simulink model "simulinkModel"  (R2015a)
settings: Solver=ode45  StartTime=0.0  StopTime=10.0  RelTol=1e-3
values from neighbouring files (symbols this model uses):
  CL0 = 0    [loadModel_EB.m]
  CLa = 22    [loadModel_EB.m]
  Cm0 = 0    [loadModel_EB.m]
  Cma = 75    [loadModel_EB.m]
  g = [gx;gextra]    [getRigidBodySS.m]
  m = sum(dm)    [getRigidBodySS.m]
  rho = 1.21    [loadModel_EB.m]
  theta0 = double(theta0)    [getRigidBodySS.m]
  xCM = (1-0.84)*total_length    (= 0.784)    [loadModel_EB.m]
undefined symbols (not defined in the file or in its folder): gamma0, ICG, Lref, Sref, theta_dot0, V0, x0, xCG, z0
libraries: simulink_extras x2, aerolib3dof2 x1, aerolibasang x1
settings Model: Creator=anatole  LastModifiedBy=anatole

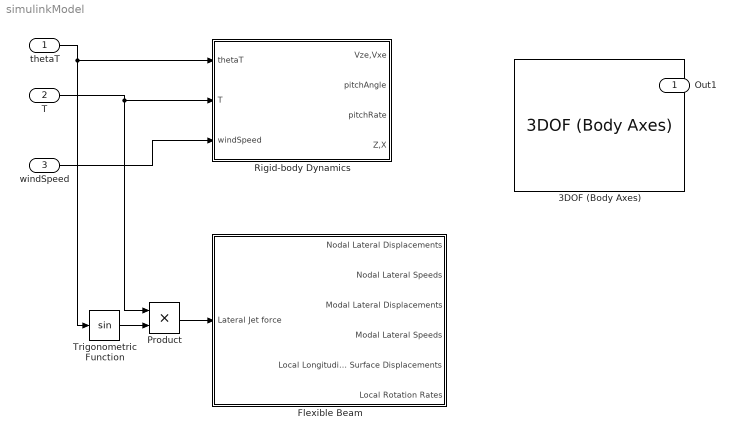
== system simulinkModel ==
  thetaT : Inport
  T : Inport  Port=2
  windSpeed : Inport  Port=3
  3DOF (Body Axes) : aerolib3dof2/3DOF (Body Axes)  units=Metric (MKS)  mtype=Fixed  v_ini=100  theta_ini=0  alpha_ini=0  q_ini=0  pos_ini=[0 0]  mass=1.0  mass_e=0.5  mass_f=3.0  Iyy=1.0  Iyy_e=0.5  Iyy_f=3.0  g_in=External  g=9.81  vre_flag=on
  Flexible Beam : Subsystem
  Product : Product
  Rigid-body Dynamics : Subsystem
  Trigonometric Function : Trigonometry
  Out1 : Outport
  wires:
  T/1 -> Product/1, Rigid-body Dynamics/2(T)
  thetaT/1 -> Trigonometric Function/1, Rigid-body Dynamics/1(thetaT)
  windSpeed/1 -> Rigid-body Dynamics/3(windSpeed)
  Product/1 -> Flexible Beam/1(Lateral Jet force)
  Trigonometric Function/1 -> Product/2

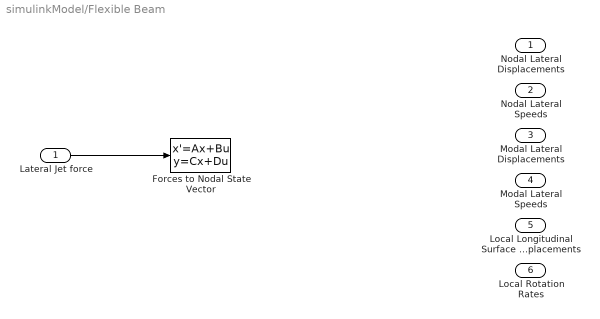
== system simulinkModel/Flexible Beam ==
  Lateral Jet force : Inport
  Forces to Nodal State Vector : StateSpace  X0=0
  Nodal Lateral Displacements : Outport
  Nodal Lateral Speeds : Outport  Port=2
  Modal Lateral Displacements : Outport  Port=3
  Modal Lateral Speeds : Outport  Port=4
  Local Longitudinal Surface Displacements : Outport  Port=5
  Local Rotation Rates : Outport  Port=6
  wires:
  Lateral Jet force/1 -> Forces to Nodal State Vector/1

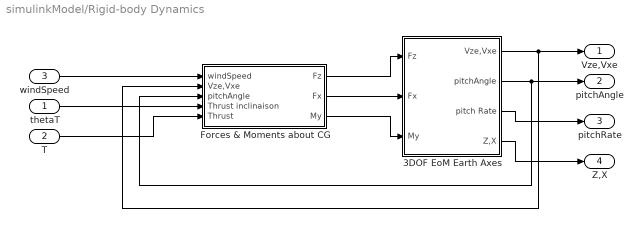
== system simulinkModel/Rigid-body Dynamics ==
  thetaT : Inport
  T : Inport  Port=2
  windSpeed : Inport  Port=3
  3DOF EoM Earth Axes : Subsystem
  Forces & Moments about CG : Subsystem
  Vze,Vxe : Outport
  pitchAngle : Outport  Port=2
  pitchRate : Outport  Port=3
  Z,X : Outport  Port=4
  wires:
  windSpeed/1 -> Forces & Moments about CG/1(windSpeed)
  3DOF EoM Earth Axes/1(Vze,Vxe) -> Forces & Moments about CG/2(Vze,Vxe), Vze,Vxe/1
  3DOF EoM Earth Axes/2(pitchAngle) -> pitchAngle/1, Forces & Moments about CG/3(pitchAngle)
  thetaT/1 -> Forces & Moments about CG/4(Thrust inclinaison)
  T/1 -> Forces & Moments about CG/5(Thrust)
  Forces & Moments about CG/3("My ") -> 3DOF EoM Earth Axes/3(My)
  Forces & Moments about CG/1(Fz) -> 3DOF EoM Earth Axes/1(Fz)
  Forces & Moments about CG/2(Fx) -> 3DOF EoM Earth Axes/2(Fx)
  3DOF EoM Earth Axes/3(pitch Rate) -> pitchRate/1
  3DOF EoM Earth Axes/4(Z,X) -> Z,X/1

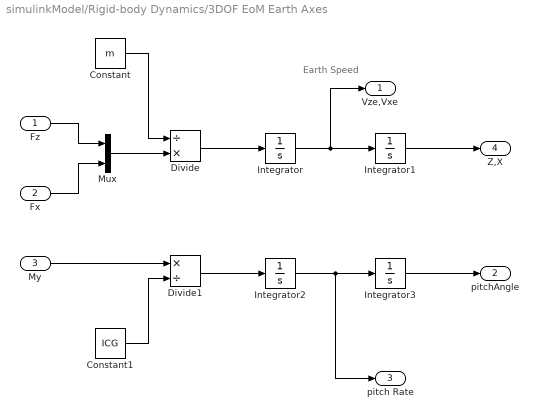
== system simulinkModel/Rigid-body Dynamics/3DOF EoM Earth Axes ==
  note: Earth Speed
  Fz : Inport
  Fx : Inport  Port=2
  My : Inport  Port=3
  Constant : Constant  Value=m
  Constant1 : Constant  Value=ICG
  Divide : Product  Inputs=/*
  Divide1 : Product  Inputs=*/
  Integrator : Integrator  InitialCondition=[-V0*sin(gamma0), V0*cos(gamma0)]
  Integrator1 : Integrator  InitialCondition=[z0, x0]
  Integrator2 : Integrator  InitialCondition=theta_dot0
  Integrator3 : Integrator  InitialCondition=theta0
  Mux : Mux  Inputs=2
  Vze,Vxe : Outport
  pitchAngle : Outport  Port=2
  pitch Rate : Outport  Port=3
  Z,X : Outport  Port=4
  wires:
  Fz/1 -> Mux/1
  Fx/1 -> Mux/2
  Mux/1 -> Divide/2
  Constant/1 -> Divide/1
  Divide/1 -> Integrator/1
  Integrator/1 -> Vze,Vxe/1, Integrator1/1
  My/1 -> Divide1/1
  Constant1/1 -> Divide1/2
  Integrator2/1 -> pitch Rate/1, Integrator3/1
  Divide1/1 -> Integrator2/1
  Integrator3/1 -> pitchAngle/1
  Integrator1/1 -> Z,X/1

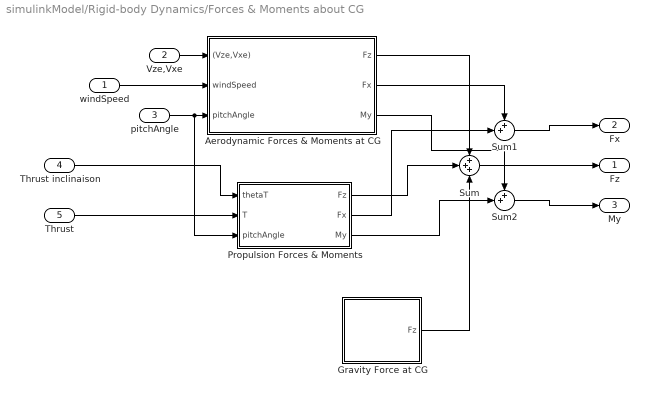
== system simulinkModel/Rigid-body Dynamics/Forces & Moments about CG ==
  windSpeed : Inport
  Vze,Vxe : Inport  Port=2
  pitchAngle : Inport  Port=3
  Thrust inclinaison : Inport  Port=4
  Thrust : Inport  Port=5
  Aerodynamic Forces & Moments at CG : Subsystem
  Gravity Force at CG : Subsystem
  Propulsion Forces & Moments : Subsystem
  Sum : Sum  Inputs=+++
  Sum1 : Sum  Inputs=++|
  Sum2 : Sum  Inputs=++|
  Fz : Outport
  Fx : Outport  Port=2
  "My " : Outport  Port=3
  wires:
  pitchAngle/1 -> Propulsion Forces & Moments/3(pitchAngle), Aerodynamic Forces & Moments at CG/3(pitchAngle)
  Propulsion Forces & Moments/3(My) -> Sum2/2
  Propulsion Forces & Moments/1(Fz) -> Sum/2
  windSpeed/1 -> Aerodynamic Forces & Moments at CG/2(windSpeed)
  Vze,Vxe/1 -> Aerodynamic Forces & Moments at CG/1((Vze,Vxe))
  Gravity Force at CG/1(Fz) -> Sum/3
  Propulsion Forces & Moments/2(Fx) -> Sum1/2
  Aerodynamic Forces & Moments at CG/3(My) -> Sum2/1
  Thrust/1 -> Propulsion Forces & Moments/2(T)
  Aerodynamic Forces & Moments at CG/1(Fz) -> Sum/1
  Aerodynamic Forces & Moments at CG/2(Fx) -> Sum1/1
  Sum/1 -> Fz/1
  Sum2/1 -> "My "/1
  Sum1/1 -> Fx/1
  Thrust inclinaison/1 -> Propulsion Forces & Moments/1(thetaT)

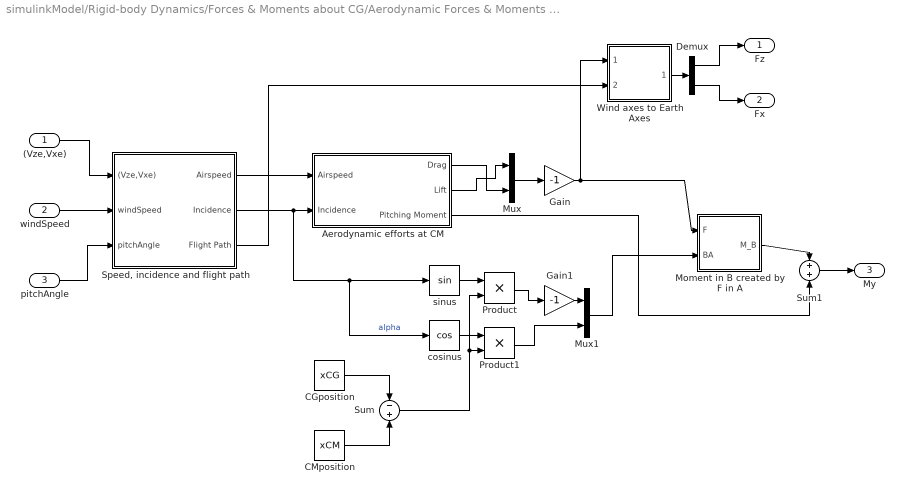
== system simulinkModel/Rigid-body Dynamics/Forces & Moments about CG/Aerodynamic Forces & Moments at CG ==
  (Vze,Vxe) : Inport
  windSpeed : Inport  Port=2
  pitchAngle : Inport  Port=3
  Aerodynamic efforts at CM : Subsystem
  CGposition : Constant  Value=xCG
  CMposition : Constant  Value=xCM
  Demux : Demux  Outputs=2
  Gain : Gain  Gain=-1
  Gain1 : Gain  Gain=-1
  Moment in B created by F in A : Subsystem
  Mux : Mux  Inputs=2
  Mux1 : Mux  Inputs=2
  Product : Product
  Product1 : Product
  "Speed, incidence and flight path" : Subsystem
  Sum : Sum  Inputs=-+
  Sum1 : Sum
  Wind axes to Earth Axes : Subsystem
  cosinus : Trigonometry  Operator=cos
  sinus : Trigonometry
  Fz : Outport
  Fx : Outport  Port=2
  My : Outport  Port=3
  wires:
  windSpeed/1 -> "Speed, incidence and flight path"/2(windSpeed)
  (Vze,Vxe)/1 -> "Speed, incidence and flight path"/1((Vze,Vxe))
  pitchAngle/1 -> "Speed, incidence and flight path"/3(pitchAngle)
  "Speed, incidence and flight path"/1(Airspeed) -> Aerodynamic efforts at CM/1(Airspeed)
  "Speed, incidence and flight path"/2(Incidence) -> cosinus/1, sinus/1, Aerodynamic efforts at CM/2(Incidence)  "alpha"
  Aerodynamic efforts at CM/2(Lift) -> Mux/1
  Aerodynamic efforts at CM/1(Drag) -> Mux/2
  Mux/1 -> Gain/1
  CGposition/1 -> Sum/1
  CMposition/1 -> Sum/2
  sinus/1 -> Product/1
  cosinus/1 -> Product1/1
  Sum/1 -> Product/2, Product1/2
  Product1/1 -> Mux1/2
  Product/1 -> Gain1/1
  Gain1/1 -> Mux1/1
  Mux1/1 -> Moment in B created by F in A/2(BA)
  Gain/1 -> Moment in B created by F in A/1(F), Wind axes to Earth Axes/1(vec_w)
  Sum1/1 -> My/1
  Aerodynamic efforts at CM/3(Pitching Moment) -> Sum1/2
  Moment in B created by F in A/1(M_B) -> Sum1/1
  "Speed, incidence and flight path"/3(Flight Path) -> Wind axes to Earth Axes/2(gamma)
  Wind axes to Earth Axes/1(vec_e) -> Demux/1
  Demux/1 -> Fz/1
  Demux/2 -> Fx/1

== system simulinkModel/Rigid-body Dynamics/Forces & Moments about CG/Gravity Force at CG ==
  Constant : Constant  Value=m*g
  Fz : Outport
  wires:
  Constant/1 -> Fz/1

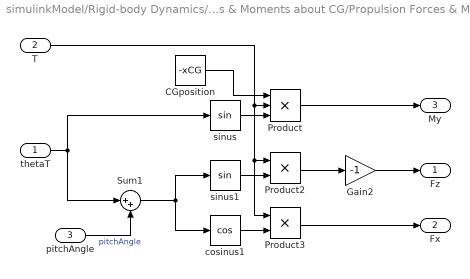
== system simulinkModel/Rigid-body Dynamics/Forces & Moments about CG/Propulsion Forces & Moments ==
  thetaT : Inport
  T : Inport  Port=2
  pitchAngle : Inport  Port=3
  CGposition : Constant  Value=-xCG
  Gain2 : Gain  Gain=-1
  Product : Product  Inputs=3
  Product2 : Product
  Product3 : Product
  Sum1 : Sum  Inputs=|++
  cosinus1 : Trigonometry  Operator=cos
  sinus : Trigonometry
  sinus1 : Trigonometry
  Fz : Outport
  Fx : Outport  Port=2
  My : Outport  Port=3
  wires:
  pitchAngle/1 -> Sum1/2  "pitchAngle"
  CGposition/1 -> Product/1
  T/1 -> Product/2, Product3/1, Product2/1
  sinus1/1 -> Product2/2
  cosinus1/1 -> Product3/2
  thetaT/1 -> sinus/1, Sum1/1
  Sum1/1 -> cosinus1/1, sinus1/1
  Product2/1 -> Gain2/1
  Gain2/1 -> Fz/1
  Product3/1 -> Fx/1
  sinus/1 -> Product/3
  Product/1 -> My/1

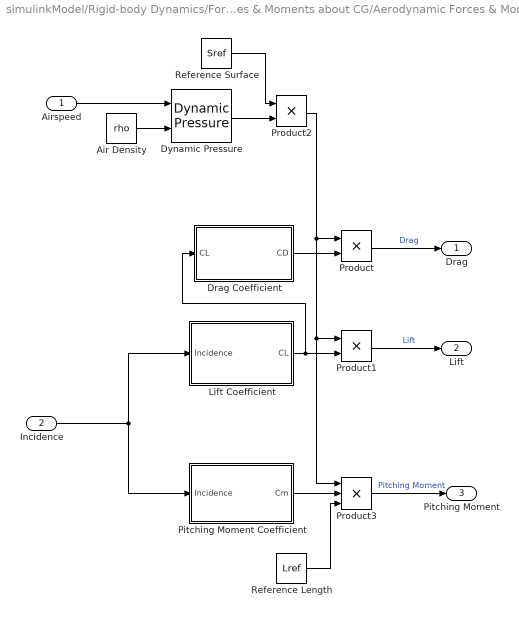
== system simulinkModel/Rigid-body Dynamics/Forces & Moments about CG/Aerodynamic Forces & Moments at CG/Aerodynamic efforts at CM ==
  Airspeed : Inport
  Incidence : Inport  Port=2
  Air Density : Constant  Value=rho
  Drag Coefficient : Subsystem
  Dynamic Pressure : aerolibasang/Dynamic Pressure
  Lift Coefficient : Subsystem
  Pitching Moment Coefficient : Subsystem
  Product : Product
  Product1 : Product
  Product2 : Product
  Product3 : Product  Inputs=3
  Reference Length : Constant  Value=Lref
  Reference Surface : Constant  Value=Sref
  Drag : Outport
  Lift : Outport  Port=2
  Pitching Moment : Outport  Port=3
  wires:
  Product1/1 -> Lift/1  "Lift"
  Product2/1 -> Product1/1, Product3/1, Product/1
  Reference Surface/1 -> Product2/1
  Drag Coefficient/1(CD) -> Product/2
  Lift Coefficient/1(CL) -> Product1/2, Drag Coefficient/1(CL)
  Dynamic Pressure/1 -> Product2/2
  Pitching Moment Coefficient/1(Cm) -> Product3/2
  Incidence/1 -> Lift Coefficient/1(Incidence), Pitching Moment Coefficient/1(Incidence)
  Product3/1 -> Pitching Moment/1  "Pitching Moment"
  Air Density/1 -> Dynamic Pressure/2
  Product/1 -> Drag/1  "Drag"
  Reference Length/1 -> Product3/3
  Airspeed/1 -> Dynamic Pressure/1

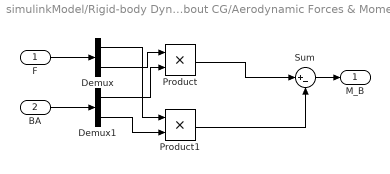
== system simulinkModel/Rigid-body Dynamics/Forces & Moments about CG/Aerodynamic Forces & Moments at CG/Moment in B created by F in A ==
  F : Inport
  BA : Inport  Port=2
  Demux : Demux  Outputs=2
  Demux1 : Demux  Outputs=2
  Product : Product
  Product1 : Product
  Sum : Sum  Inputs=|+-
  M_B : Outport
  wires:
  BA/1 -> Demux1/1
  F/1 -> Demux/1
  Demux1/1 -> Product/2
  Demux/2 -> Product/1
  Demux1/2 -> Product1/2
  Demux/1 -> Product1/1
  Product1/1 -> Sum/2
  Sum/1 -> M_B/1
  Product/1 -> Sum/1

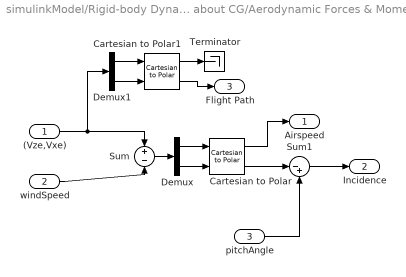
== system simulinkModel/Rigid-body Dynamics/Forces & Moments about CG/Aerodynamic Forces & Moments at CG/Speed, incidence and flight path ==
  (Vze,Vxe) : Inport
  windSpeed : Inport  Port=2
  pitchAngle : Inport  Port=3
  Cartesian to Polar : simulink_extras/Transformations/Cartesian to Polar
  Cartesian to Polar1 : simulink_extras/Transformations/Cartesian to Polar
  Demux : Demux  Outputs=2
  Demux1 : Demux  Outputs=2
  Sum : Sum  Inputs=+-
  Sum1 : Sum  Inputs=|-+
  Terminator : Terminator
  Airspeed : Outport
  Incidence : Outport  Port=2
  Flight Path : Outport  Port=3
  wires:
  windSpeed/1 -> Sum/2
  Sum/1 -> Demux/1
  Demux/1 -> Cartesian to Polar/1
  Demux/2 -> Cartesian to Polar/2
  pitchAngle/1 -> Sum1/2
  Cartesian to Polar/2 -> Sum1/1
  Sum1/1 -> Incidence/1
  Cartesian to Polar/1 -> Airspeed/1
  (Vze,Vxe)/1 -> Demux1/1, Sum/1
  Demux1/1 -> Cartesian to Polar1/1
  Demux1/2 -> Cartesian to Polar1/2
  Cartesian to Polar1/1 -> Terminator/1
  Cartesian to Polar1/2 -> Flight Path/1

== system simulinkModel/Rigid-body Dynamics/Forces & Moments about CG/Aerodynamic Forces & Moments at CG/Wind axes to Earth Axes ==
  vec_w : Inport
  gamma : Inport  Port=2
  MATLAB Function : MATLAB Function  TreatAsAtomicUnit=on
  vec_e : Outport
  wires:
  vec_w/1 -> MATLAB Function/1(vec1)
  gamma/1 -> MATLAB Function/2(gamma)
  MATLAB Function/1(vec2) -> vec_e/1

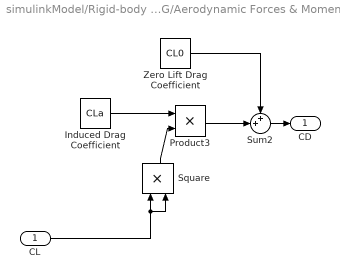
== system simulinkModel/Rigid-body Dynamics/Forces & Moments about CG/Aerodynamic Forces & Moments at CG/Aerodynamic efforts at CM/Drag Coefficient ==
  CL : Inport
  Induced Drag Coefficient : Constant  Value=CLa
  Product3 : Product
  Square : Product
  Sum2 : Sum  Inputs=++|
  Zero Lift Drag Coefficient : Constant  Value=CL0
  CD : Outport
  wires:
  Zero Lift Drag Coefficient/1 -> Sum2/1
  Product3/1 -> Sum2/2
  Square/1 -> Product3/2
  CL/1 -> Square/2, Square/1
  Induced Drag Coefficient/1 -> Product3/1
  Sum2/1 -> CD/1

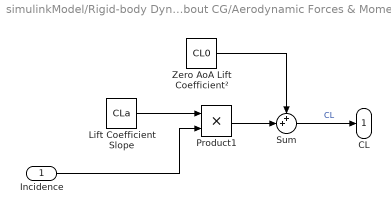
== system simulinkModel/Rigid-body Dynamics/Forces & Moments about CG/Aerodynamic Forces & Moments at CG/Aerodynamic efforts at CM/Lift Coefficient ==
  Incidence : Inport
  Lift Coefficient Slope : Constant  Value=CLa
  Product1 : Product
  Sum : Sum  Inputs=++|
  Zero AoA Lift Coefficient² : Constant  Value=CL0
  CL : Outport
  wires:
  Sum/1 -> CL/1  "CL"
  Incidence/1 -> Product1/2
  Lift Coefficient Slope/1 -> Product1/1
  Product1/1 -> Sum/2
  Zero AoA Lift Coefficient²/1 -> Sum/1

== system simulinkModel/Rigid-body Dynamics/Forces & Moments about CG/Aerodynamic Forces & Moments at CG/Aerodynamic efforts at CM/Pitching Moment Coefficient ==
  Incidence : Inport
  Pitching Moment Coeff Slope : Constant  Value=Cma
  Product2 : Product
  Sum1 : Sum  Inputs=++|
  Zero AoA Pitching Moment Coeff : Constant  Value=Cm0
  Cm : Outport
  wires:
  Product2/1 -> Sum1/2
  Zero AoA Pitching Moment Coeff/1 -> Sum1/1
  Pitching Moment Coeff Slope/1 -> Product2/1
  Sum1/1 -> Cm/1
  Incidence/1 -> Product2/2

== matlab function simulinkModel/Rigid-body Dynamics/Forces & Moments about CG/Aerodynamic Forces & Moments at CG/Wind axes to Earth Axes/MATLAB Function ==
  data: vec1 input; vec2 output; gamma input
function vec2 = fcn(vec1,gamma)


A = [cos(gamma) -sin(gamma); sin(gamma) cos(gamma)];
vec2 = A*vec1;
